simulink model "model3_simulink"  (R2025b)
settings: Solver=ode45  StartTime=0.0  StopTime=200  RelTol=1e-3
undefined symbols (not defined in the file): alpha, B, Kd1, Kd2, Ki1, Ki2, Kp1, Kp2, Kps, Tg, TieGain, Tps, Tt
libraries: slpidlib x2, simulink x1, fuzblock x1
settings Model: Creator=parth  LastModifiedBy=parth

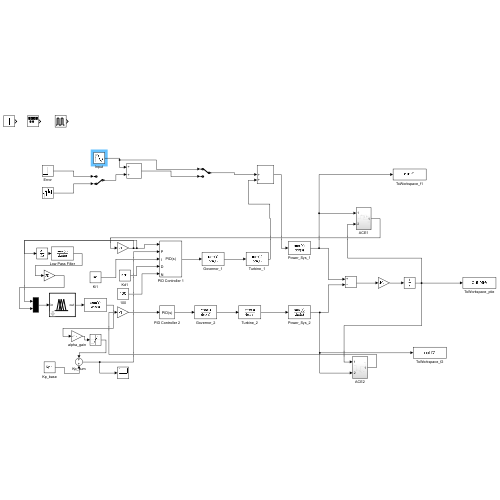
[thumbnail: Simulink's stored preview of the top-level diagram]
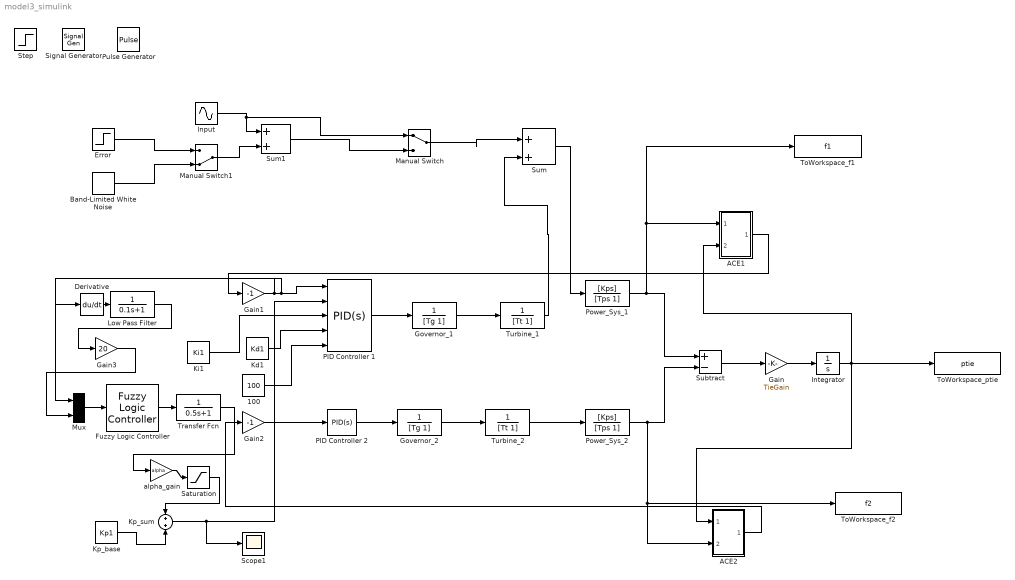
== system model3_simulink ==
  100 : Constant  Value=100
  ACE1 : Subsystem
  ACE2 : Subsystem
  Band-Limited White Noise : simulink/Sources/Band-Limited White Noise  Cov=1e-5  Ts=0.01  seed=[23341]
  Derivative : Derivative
  Error : Step  Time=40  After=0.02  SampleTime=0
  Fuzzy Logic Controller : fuzblock/Fuzzy Logic  Controller  FIS=fuzzy_pid  OutputSampleNumber=101  DataType=double  UseLookupTable=off  NumBreakpoints=10  FuzzifiedInputs=off  RuleFiringStrengths=off  RuleOutputs=off  AggregatedOutputs=off  SimulateUsing=Code generation  OutOfRangeInputValueMessage=warning  NoRuleFiredMessage=warning  EmptyOutputFuzzySetMessage=warning
  Gain : Gain  Gain=TieGain
  Gain1 : Gain  Gain=-1
  Gain2 : Gain  Gain=-1
  Gain3 : Gain  Gain=20
  Governor_1 : TransferFcn  Denominator=[Tg 1]
  Governor_2 : TransferFcn  Denominator=[Tg 1]
  Input : Sin  Amplitude=0.01  Frequency=0.1  SampleTime=0
  Integrator : Integrator
  Kd1 : Constant  Value=Kd1
  Ki1 : Constant  Value=Ki1
  Kp_base : Constant  Value=Kp1
  Kp_sum : Sum
  Low Pass Filter : TransferFcn  Denominator=[0.1 1]
  Manual Switch : ManualSwitch
  Manual Switch1 : ManualSwitch  CurrentSetting=0
  Mux : Mux  Inputs=2
  PID Controller 1 : slpidlib/PID Controller  Controller=PID  Form=Parallel  TimeDomain=Continuous-time  UseExternalTs=off  SampleTime=-1  IntegratorMethod=Forward Euler  FilterMethod=Forward Euler  ControllerParametersSource=external  P=Kp1  I=Ki1  UseKiTs=off  D=Kd1  UseExternalDerivativeSource=off  N=100  UseFilter=on  TunerSelectOption=Frequency Response Based  InitialConditionSource=internal  InitialConditionForIntegrator=0  InitialConditionForFilter=0  DifferentiatorICPrevScaledInput=0  ExternalReset=none  TrackingMode=off  Kt=1  LimitOutput=off  SatLimitsSource=internal  UpperSaturationLimit=inf  LowerSaturationLimit=-inf  LinearizeAsGain=on  AntiWindupMode=none  Kb=1  LimitIntegrator=off  UpperIntegratorSaturationLimit=inf  LowerIntegratorSaturationLimit=-inf  POutMin=[]  POutMax=[]  IOutMin=[]  IOutMax=[]  DOutMin=[]  DOutMax=[]  NOutMin=[]  NOutMax=[]  SumOutMin=[]  SumOutMax=[]  SaturationOutMin=[]  SaturationOutMax=[]  PParamMin=[]  PParamMax=[]  IParamMin=[]  IParamMax=[]  DParamMin=[]  DParamMax=[]  NParamMin=[]  NParamMax=[]  KbParamMin=[]  KbParamMax=[]  KtParamMin=[]  KtParamMax=[]  KbOutMin=[]  KbOutMax=[]  KtOutMin=[]  KtOutMax=[]  IntegratorOutMin=[]  IntegratorOutMax=[]  FilterOutMin=[]  FilterOutMax=[]  SumI1OutMin=[]  SumI1OutMax=[]  SumI2OutMin=[]  SumI2OutMax=[]  SumI3OutMin=[]  SumI3OutMax=[]  SumI4OutMin=[]  SumI4OutMax=[]  SumDOutMin=[]  SumDOutMax=[]  DifferentiatorOutMin=[]  DifferentiatorOutMax=[]  FilterDiffOutCoefMin=[]  FilterDiffOutCoefMax=[]  ReciprocalOutMin=[]  ReciprocalOutMax=[]  SumDenOutMin=[]  SumDenOutMax=[]  SumNumOutMin=[]  SumNumOutMax=[]  DivideOutMin=[]  DivideOutMax=[]  UdiffTsProdOutMin=[]  UdiffTsProdOutMax=[]  NTsProdOutMin=[]  NTsProdOutMax=[]  UintegralTsProdOutMin=[]  UintegralTsProdOutMax=[]  UngainTsProdOutMin=[]  UngainTsProdOutMax=[]  ClampingZeroOutDataTypeStr=Inherit: Inherit via back propagation  ClampingZeroOutMin=[]  ClampingZeroOutMax=[]  FilterDenConstantOutDataTypeStr=Inherit: Inherit via back propagation  FilterDenConstantOutMin=[]  FilterDenConstantOutMax=[]  PCopyOutDataTypeStr=Inherit: Inherit via back propagation  PCopyOutMin=[]  PCopyOutMax=[]  NCopyOutDataTypeStr=Inherit: Inherit via back propagation  NCopyOutMin=[]  NCopyOutMax=[]  IntegratorContinuousStateAttributes=''  IntegratorStateMustResolveToSignalObject=off  IntegratorRTWStateStorageClass=Auto  FilterContinuousStateAttributes=''  FilterStateMustResolveToSignalObject=off  FilterRTWStateStorageClass=Auto  ParallelPVariant=ExternalParameters  IdealPVariant=Disabled  IVariant=ExternalParameters  DVariant=ExternalParameters  IntegratorVariant=Continuous  SatVariant=Disabled  AWVariant=Passthrough  PCopyVariant=Disabled  TRVariant=Disabled  FdbkBlocksVariant=Forward  IdealPFdbkVariant=Disabled  SatFdbkVariant=Disabled  DerivativeFilterVariant=ContFilter  NVariant=ExternalParameters  NCopyVariant=Disabled  FilterICVariant=InternalICsFilter  IntegratorICVariant=InternalICs  ExternalResetVariant=Disabled  TRSumVariant=Passthrough  SumFdbkVariant=Disabled  SumVariant=Sum_PID  TsampFilterVariant=InternalTs  TsampNgainVariant=Passthrough  TsampIntegralVariant=Disabled_SignalSpec  ExternalSaturationOutDataTypeStr=Inherit: Same as second input  DerivativeSourceVariant=ErrorSignal  PreIntVariant=InternalPreInt
  PID Controller 2 : slpidlib/PID Controller  Controller=PID  Form=Parallel  TimeDomain=Continuous-time  UseExternalTs=off  SampleTime=-1  IntegratorMethod=Forward Euler  FilterMethod=Forward Euler  ControllerParametersSource=internal  P=Kp2  I=Ki2  UseKiTs=off  D=Kd2  UseExternalDerivativeSource=off  N=100  UseFilter=on  TunerSelectOption=Frequency Response Based  InitialConditionSource=internal  InitialConditionForIntegrator=0  InitialConditionForFilter=0  DifferentiatorICPrevScaledInput=0  ExternalReset=none  TrackingMode=off  Kt=1  LimitOutput=off  SatLimitsSource=internal  UpperSaturationLimit=inf  LowerSaturationLimit=-inf  LinearizeAsGain=on  AntiWindupMode=none  Kb=1  LimitIntegrator=off  UpperIntegratorSaturationLimit=inf  LowerIntegratorSaturationLimit=-inf  POutMin=[]  POutMax=[]  IOutMin=[]  IOutMax=[]  DOutMin=[]  DOutMax=[]  NOutMin=[]  NOutMax=[]  SumOutMin=[]  SumOutMax=[]  SaturationOutMin=[]  SaturationOutMax=[]  PParamMin=[]  PParamMax=[]  IParamMin=[]  IParamMax=[]  DParamMin=[]  DParamMax=[]  NParamMin=[]  NParamMax=[]  KbParamMin=[]  KbParamMax=[]  KtParamMin=[]  KtParamMax=[]  KbOutMin=[]  KbOutMax=[]  KtOutMin=[]  KtOutMax=[]  IntegratorOutMin=[]  IntegratorOutMax=[]  FilterOutMin=[]  FilterOutMax=[]  SumI1OutMin=[]  SumI1OutMax=[]  SumI2OutMin=[]  SumI2OutMax=[]  SumI3OutMin=[]  SumI3OutMax=[]  SumI4OutMin=[]  SumI4OutMax=[]  SumDOutMin=[]  SumDOutMax=[]  DifferentiatorOutMin=[]  DifferentiatorOutMax=[]  FilterDiffOutCoefMin=[]  FilterDiffOutCoefMax=[]  ReciprocalOutMin=[]  ReciprocalOutMax=[]  SumDenOutMin=[]  SumDenOutMax=[]  SumNumOutMin=[]  SumNumOutMax=[]  DivideOutMin=[]  DivideOutMax=[]  UdiffTsProdOutMin=[]  UdiffTsProdOutMax=[]  NTsProdOutMin=[]  NTsProdOutMax=[]  UintegralTsProdOutMin=[]  UintegralTsProdOutMax=[]  UngainTsProdOutMin=[]  UngainTsProdOutMax=[]  ClampingZeroOutDataTypeStr=Inherit: Inherit via back propagation  ClampingZeroOutMin=[]  ClampingZeroOutMax=[]  FilterDenConstantOutDataTypeStr=Inherit: Inherit via back propagation  FilterDenConstantOutMin=[]  FilterDenConstantOutMax=[]  PCopyOutDataTypeStr=Inherit: Inherit via back propagation  PCopyOutMin=[]  PCopyOutMax=[]  NCopyOutDataTypeStr=Inherit: Inherit via back propagation  NCopyOutMin=[]  NCopyOutMax=[]  IntegratorContinuousStateAttributes=''  IntegratorStateMustResolveToSignalObject=off  IntegratorRTWStateStorageClass=Auto  FilterContinuousStateAttributes=''  FilterStateMustResolveToSignalObject=off  FilterRTWStateStorageClass=Auto  ParallelPVariant=InternalParameters  IdealPVariant=Disabled  IVariant=InternalParameters  DVariant=InternalParameters  IntegratorVariant=Continuous  SatVariant=Disabled  AWVariant=Passthrough  PCopyVariant=Disabled  TRVariant=Disabled  FdbkBlocksVariant=Forward  IdealPFdbkVariant=Disabled  SatFdbkVariant=Disabled  DerivativeFilterVariant=ContFilter  NVariant=InternalParameters  NCopyVariant=Disabled  FilterICVariant=InternalICsFilter  IntegratorICVariant=InternalICs  ExternalResetVariant=Disabled  TRSumVariant=Passthrough  SumFdbkVariant=Disabled  SumVariant=Sum_PID  TsampFilterVariant=InternalTs  TsampNgainVariant=Passthrough  TsampIntegralVariant=Disabled_SignalSpec  ExternalSaturationOutDataTypeStr=Inherit: Same as second input  DerivativeSourceVariant=ErrorSignal  PreIntVariant=InternalPreInt
  Power_Sys_1 : TransferFcn  Numerator=[Kps]  Denominator=[Tps 1]
  Power_Sys_2 : TransferFcn  Numerator=[Kps]  Denominator=[Tps 1]
  Pulse Generator : DiscretePulseGenerator  PulseType=Time based  Amplitude=0.01  Period=1000  PhaseDelay=10
  Saturation : Saturate
  Scope1 : Scope
      settings: ActiveDisplayYMinimum=-1  ActiveDisplayYMaximum=1
  Signal Generator : SignalGenerator  WaveForm=square  Amplitude=0.01  Frequency=0.05  Units=rad/sec
  Step : Step  After=0.01  SampleTime=0  VectorParams1D=off
  Subtract : Sum  Inputs=+-
  Sum : Sum  Inputs=|++
  Sum1 : Sum
  ToWorkspace_f1 : ToWorkspace  VariableName=f1  SampleTime=-1
      settings: Save2DSignal=2-D array (concatenate along first dimension)
  ToWorkspace_f2 : ToWorkspace  VariableName=f2  SampleTime=-1
      settings: Save2DSignal=2-D array (concatenate along first dimension)
  ToWorkspace_ptie : ToWorkspace  VariableName=ptie  SampleTime=-1
      settings: Save2DSignal=2-D array (concatenate along first dimension)
  Transfer Fcn : TransferFcn  Denominator=[0.5 1]
  Turbine_1 : TransferFcn  Denominator=[Tt 1]
  Turbine_2 : TransferFcn  Denominator=[Tt 1]
  alpha_gain : Gain  Gain=alpha
  wires:
  Turbine_1/1 -> Sum/2
  PID Controller 2/1 -> Governor_2/1
  Turbine_2/1 -> Power_Sys_2/1
  Sum1/1 -> Manual Switch/2
  Gain/1 -> Integrator/1
  Power_Sys_2/1 -> ToWorkspace_f2/1, ACE2/2(In2), Subtract/2
  Power_Sys_1/1 -> ToWorkspace_f1/1, ACE1/1(In1), Subtract/1
  Gain2/1 -> PID Controller 2/1
  Subtract/1 -> Gain/1
  Band-Limited White Noise/1 -> Manual Switch1/2
  Error/1 -> Manual Switch1/1
  ACE2/1(Out1) -> Gain2/1
  Governor_2/1 -> Turbine_2/1
  PID Controller 1/1 -> Governor_1/1
  Manual Switch/1 -> Sum/1
  ACE1/1(Out1) -> Gain1/1
  Input/1 -> Manual Switch/1, Sum1/1
  Manual Switch1/1 -> Sum1/2
  Sum/1 -> Power_Sys_1/1
  Governor_1/1 -> Turbine_1/1
  Gain1/1 -> Mux/1, Derivative/1, PID Controller 1/1
  Integrator/1 -> ACE1/2(In2), ToWorkspace_ptie/1, ACE2/1(In1)
  Ki1/1 -> PID Controller 1/3
  Kd1/1 -> PID Controller 1/4
  100/1 -> PID Controller 1/5
  Mux/1 -> Fuzzy Logic Controller/1
  Derivative/1 -> Low Pass Filter/1
  Low Pass Filter/1 -> Gain3/1
  Gain3/1 -> Mux/2
  Kp_base/1 -> Kp_sum/2
  Kp_sum/1 -> Scope1/1, PID Controller 1/2
  alpha_gain/1 -> Saturation/1
  Saturation/1 -> Kp_sum/1
  Fuzzy Logic Controller/1 -> Transfer Fcn/1
  Transfer Fcn/1 -> alpha_gain/1

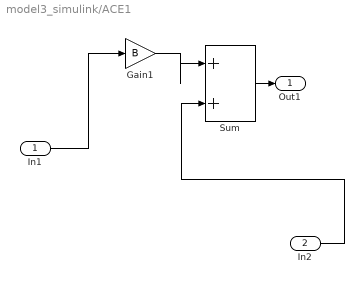
== system model3_simulink/ACE1 ==
  In1 : Inport
  In2 : Inport  Port=2
  Gain1 : Gain  Gain=B
  Sum : Sum  Inputs=|++
  Out1 : Outport
  wires:
  In1/1 -> Gain1/1
  Gain1/1 -> Sum/1
  Sum/1 -> Out1/1
  In2/1 -> Sum/2

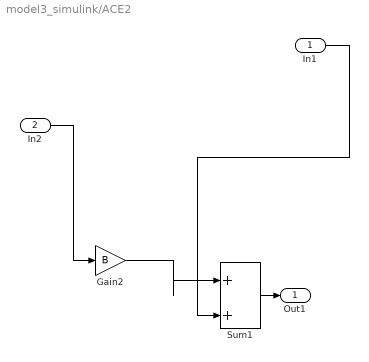
== system model3_simulink/ACE2 ==
  In1 : Inport
  In2 : Inport  Port=2
  Gain2 : Gain  Gain=B
  Sum1 : Sum  Inputs=|++
  Out1 : Outport
  wires:
  Gain2/1 -> Sum1/1
  In2/1 -> Gain2/1
  In1/1 -> Sum1/2
  Sum1/1 -> Out1/1
